simulink subsystem "H_bridge"  (R2020a)
settings: Solver=VariableStepAuto  StartTime=0.0  StopTime=10.0  RelTol=1e-3
values from neighbouring files (symbols this model uses):
  Vmax = 12    [define_constants.m]
libraries: simulink x1
settings Model: Creator=alex  LastModifiedBy=alex

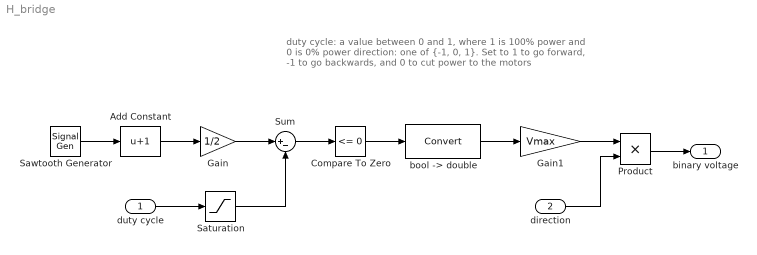
== system H_bridge ==
  note: duty cycle: a value between 0 and 1, where 1 is 100% power and 0 is 0% power
      |
      | direction: one of {-1, 0, 1}. Set to 1 to go forward, -1 to go backwards, and 0 to cut power to the motors
  duty cycle : Inport
  direction : Inport  Port=2
  Add Constant : Bias  Bias=1
  Compare To Zero : simulink/Logic and Bit Operations/Compare To Zero  relop=<=  OutDataTypeStr=boolean
  Gain : Gain  Gain=1/2
  Gain1 : Gain  Gain=Vmax
  Product : Product
  Saturation : Saturate  UpperLimit=1  LowerLimit=0
  Sawtooth Generator : SignalGenerator  WaveForm=sawtooth  Frequency=500
  Sum : Sum  Inputs=|+-
  "bool -> double" : DataTypeConversion
  binary voltage : Outport
  wires:
  Add Constant/1 -> Gain/1
  Sum/1 -> Compare To Zero/1
  "bool -> double"/1 -> Gain1/1
  Sawtooth Generator/1 -> Add Constant/1
  Gain/1 -> Sum/1
  Compare To Zero/1 -> "bool -> double"/1
  Gain1/1 -> Product/1
  Product/1 -> binary voltage/1
  direction/1 -> Product/2
  Saturation/1 -> Sum/2
  duty cycle/1 -> Saturation/1
